simulink model "Test_World_3_cs"  (R2019a)
settings: Solver=FixedStepDiscrete  StartTime=0.0  StopTime=15  FixedStep=1/300  RelTol=1e-3
PreLoadFcn:
  | mbxruntime.callbacks.PreLoadFcn(bdroot);
  | check_NUTS_defined
  | model_closed = 0;
  | assignin('base',['model_closed_' bdroot],false);
PostLoadFcn:
  | mbxruntime.callbacks.PostLoadFcn(bdroot);
InitFcn:
  | mbxruntime.callbacks.InitFcn(bdroot);
StartFcn:
  | mbxruntime.callbacks.StartFcn(bdroot);
StopFcn:
  | mbxruntime.callbacks.StopFcn(bdroot);;
  | 
model workspace: external: MAT-File .\Test_World_3_cs_hws.mat (data not in the file)
undefined symbols (not defined in the file or in its folder): AngularVelocity, Clock_, Data, Data_SL_Info, DiscIntNeverNeededParam, Encoding, Encoding_SL_Info, Header, Height, InitImageOutputDir, LinearAcceleration, Orientation, Pose, Poses, Poses_SL_Info, Position, Step, Twist, Width
libraries: robotlib x26, simulink_extras x19, PreScanSimulinkLibrary x6, PBCSimulinkLibrary x5, dspindex x4, robotcorelib x2, sharedtransform x2, visionconversions x1, visionsinks x1
(part 2 of 5)

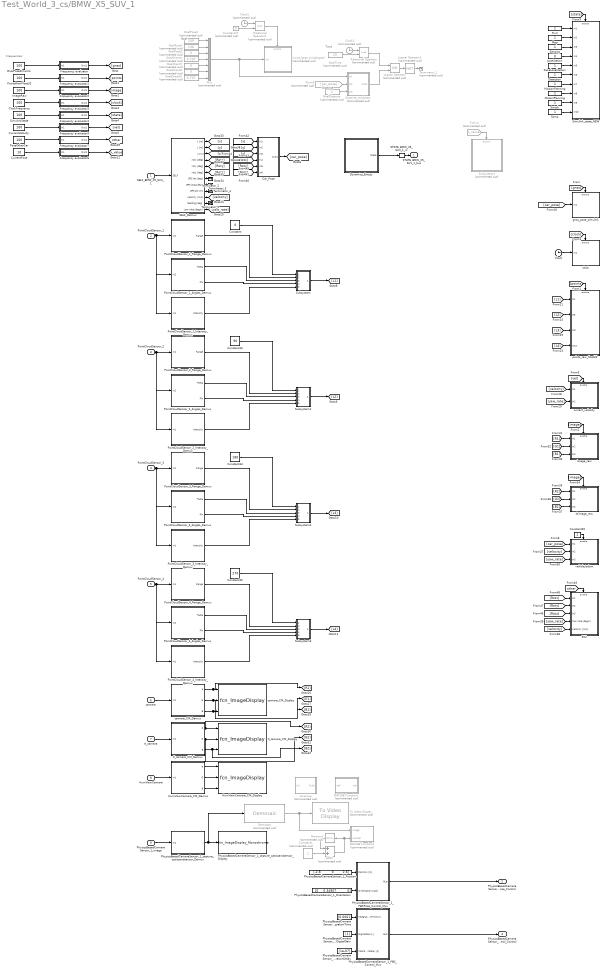
== system Test_World_3_cs/BMW_X5_SUV_1 ==
  note: Goal
  note: Distance
  note: Time
  note: Frequencies
  SELF_BMW_X5_SUV_1 : Inport  Tag=inport/SelfPort  OutDataTypeStr=Bus: PRESCAN_SELFSENSORDATA  PortDimensions=1  SampleTime=1/300  BusOutputAsStruct=on
  PointCloudSensor_1 : Inport  Tag=inport/PointCloudInport  Port=2  OutDataTypeStr=single  SampleTime=1/20  BusOutputAsStruct=on
  PointCloudSensor_2 : Inport  Tag=inport/PointCloudInport  Port=3  OutDataTypeStr=single  SampleTime=1/20  BusOutputAsStruct=on
  PointCloudSensor_3 : Inport  Tag=inport/PointCloudInport  Port=4  OutDataTypeStr=single  SampleTime=1/20  BusOutputAsStruct=on
  PointCloudSensor_4 : Inport  Tag=inport/PointCloudInport  Port=5  OutDataTypeStr=single  SampleTime=1/20  BusOutputAsStruct=on
  camera : Inport  Tag=inport/Camera/CameraSensor  Port=6  OutDataTypeStr=uint8  SampleTime=1/20  BusOutputAsStruct=on
  tl_camera : Inport  Tag=inport/Camera/CameraSensor  Port=7  OutDataTypeStr=uint8  SampleTime=1/20  BusOutputAsStruct=on
  HumViewCamera : Inport  Tag=inport/Camera/CameraSensor  Port=8  OutDataTypeStr=uint8  SampleTime=1/60  BusOutputAsStruct=on
  PhysicsBasedCameraSensor_1_image : Inport  Tag=inport/plugin/sfun_PBCOutput  Port=9  BusOutputAsStruct=on
  Add5 : Sum  Commented=on
  Car_Pose : Subsystem
  Clock : Clock
  Clock1 : Clock  Commented=on
  Clock2 : Clock  Commented=on
  ClockFrequency : Constant  Value=100
  Constant : Constant  Value=0  OutDataTypeStr=Inherit: Inherit via back propagation
  Constant1 : Constant  Commented=on  OutDataTypeStr=int32
  Constant20 : Constant
  Constant27 : Constant  Commented=on  Value=0
  Constant33 : Constant  Value=90  OutDataTypeStr=Inherit: Inherit via back propagation
  Constant34 : Constant  Value=180  OutDataTypeStr=Inherit: Inherit via back propagation
  Constant35 : Constant  Value=270  OutDataTypeStr=Inherit: Inherit via back propagation
  CurrentPose : Constant  Value=10
  CurrentVelocity : Constant  Value=100
  Demosaic : visionconversions/Demosaic  Commented=on  algorithm=Obsolete  algorithmActive=Gradient-corrected linear  alignment=BGGR  imagePorts=One multidimensional signal  roundingMode=Floor  overflowMode=on  prodOutputMode=Binary point scaling  prodOutputWordLength=32  prodOutputFracLength=10  prodOutputSlope=2^-10  accumSlope=2^-10
      settings: SourceProductName=Computer Vision Toolbox  SourceProductBaseCode=VP
  Detection : Constant
  Distance_evaluator : Subsystem  Commented=on
  Dynamics_Empty : Subsystem  Tag=Dynamics_Empty
      mask Help: eval('openHelp(202)')
      mask Display: port_label('output', 1, 'State');text(0,0,' Empty\n')
  FakeLocalization : Constant
  Frequency evaluator : Subsystem
  Frequency evaluator1 : Subsystem
  Frequency evaluator2 : Subsystem
  Frequency evaluator3 : Subsystem
  Frequency evaluator4 : Subsystem
  Frequency evaluator5 : Subsystem
  Frequency evaluator6 : Subsystem
  Frequency evaluator7 : Subsystem
  From4 : From  Commented=on  GotoTag=x_value
  From6 : From  Commented=on  GotoTag=car_pose
  GnssPoseSimulink : Constant  Value=100
  GoalDistance : Constant  Commented=on  Value=2
  GoalOrientW : Constant  Commented=on  Value=0.707
  GoalOrientX : Constant  Commented=on  Value=0.707
  GoalOrientY : Constant  Commented=on  Value=0
  GoalOrientZ : Constant  Commented=on  Value=0
  GoalPoseX : Constant  Commented=on  Value=249
  GoalPoseY : Constant  Commented=on  Value=136
  GoalPoseZ : Constant  Commented=on  Value=0
  GoalTime : Constant  Commented=on  Value=10
  HumViewCamera_CM_Demux : Subsystem  Tag=demux/Camera/Color  mask{SensorName=HumViewCamera, hres=1871, vres=1080}
      mask prompts: SensorName "Sensor Name"; hres "Horizontal Resolution"; vres "Vertical Resolution"
      mask Help: eval('openHelp(457)')
      mask Display:
      | fprintf('MONO CAMERA:\n Color\n %s \n %d x %d px',SensorName,hres,vres)
      | port_label('output',1,'R')
      | port_label('output',2,'G')
      | port_label('output',3,'B')
  HumViewCamera_CM_Display : M-S-Function  Tag=CameraSensor_Color_Display  InitFcn=InitImageOutputDir(gcb);  FunctionName=fcn_ImageDisplay  Parameters=SensorName EnableDisplay EnablePosition DisplayPosition FigureHandle SaveResults BitmapFormat TempOutputDir CameraType DataType  mask(PreScan Color Display Block){SensorName=HumViewCamera, EnableDisplay=on, EnablePosition=off, DisplayPosition=[10 10 1871 1080], FigureHandle=904007, SaveResults=off, Format=PNG, TempOutputDir=Results/SimResults_20190712_170005/HumViewCamera, CameraType=Mono, DataType=uint8}
      mask prompts: SensorName "User Specified: Title of Display"; EnableDisplay "Active"; EnablePosition "Set Display window position"; DisplayPosition "Display window position [xpos ypos width height]"; FigureHandle "Unique Handle"; SaveResults "Save results"; TempOutputDir "OutputDir"; CameraType "Camera Type"; DataType "Image Data Type"
      mask help: This block displays the RGB output of a PreScan camera sensor.
      mask init:
      | if EnableDisplay
      |     EnableString='';
      |     EnableColor='gray';
      | else
      |     EnableString='INACTIVE';
      |     EnableColor='red';
      | end
      | switch Format
      |     case 1
      |         BitmapFormat = 'png';
      |     case 2
      |         BitmapFormat = 'bmp';
      |     case 3
      |         BitmapFormat = 'jpg';
      | end 
      | if CameraType==1
      |     CameraTypeName='MONO';
      |     PortNumber=0;
      | else
      |     CameraTypeName='STEREO';
      |     PortNumber=3;
      | end
      settings: CopyFcn=CopyFcnDisplay  DeleteFcn=PreScanBlockDeleteFcn;  ModelCloseFcn=fcn_ImageDisplay_ModelCloseFcn
      mask Help: eval('openHelp(457)')
      mask Callback EnablePosition:
      | MV=get_param(gcb,'MaskVisibilities');
      | if strcmp(get_param(gcb,'EnablePosition'),'on')
      |     MV{4}='on';
      | else
      |     MV{4}='off';
      | end
      | set_param(gcb,'MaskVisibilities',MV);
      | clear MV;
      mask TypeOptions Format: PNG | BMP | JPG
      mask TypeOptions CameraType: Mono | Stereo
      mask TypeOptions DataType: uint8 | single
      mask Display:
      | color(EnableColor);
      | fprintf('%s\n DISPLAY:\n Color \n %s',EnableString,SensorName)
      | port_label('input',1,'R')
      | port_label('input',2,'G')
      | port_label('input',3,'B')
      | port_label('input',PortNumber+1,'R')
      | port_label('input',PortNumber+2,'G')
      | port_label('input',PortNumber+3,'B')
  IMU : Subsystem
  ImageRaw : Constant  Value=100
  Localization : Constant  Value=0
  Logical Operator : Logic  Commented=on  Operator=OR  AllPortsSameDT=off  OutDataTypeStr=boolean
  Logical Operator1 : Logic  Commented=on  Operator=NOT  AllPortsSameDT=off  OutDataTypeStr=boolean
  MATLAB Function1 : MATLAB Function  Commented=on  TreatAsAtomicUnit=on
  MATLAB Function2 : MATLAB Function  Commented=on  TreatAsAtomicUnit=on
  Map : Constant
  Memory2 : Memory  Commented=on  InheritSampleTime=on
  MissionPlanning : Constant
  MotionPlanning : Constant
  Mux : Mux  Commented=on  Inputs=7
  PhysicsBasedCameraSensor_1_DigitalGain : Constant  Tag=PhysicsBasedCameraSensor_1_DigitalGain  Value=[1]
  PhysicsBasedCameraSensor_1_IntegrationTime : Constant  Tag=PhysicsBasedCameraSensor_1_IntegrationTime  Value=[0.0001]
  PhysicsBasedCameraSensor_1_InterRowIntegrationDelay : Constant  Tag=PhysicsBasedCameraSensor_1_InterRowIntegrationDelay  Value=[1e-07]
  PhysicsBasedCameraSensor_1_Orientation : Constant  Tag=PhysicsBasedCameraSensor_1_Orientation  Value="[0     0.34907           0]"
  PhysicsBasedCameraSensor_1_PBCPose_Control_Mux : Subsystem  Tag=mux/plugin/PBC_TA
  PhysicsBasedCameraSensor_1_PBC_Control_Mux : Subsystem  Tag=mux/plugin/PBC_ControlSignalsBasic
  PhysicsBasedCameraSensor_1_Position : Constant  Tag=PhysicsBasedCameraSensor_1_Position  Value="[-2.8           0         2.6]"
  PhysicsBasedCameraSensor_1_capture_opticsandsensor_Demux : Subsystem  Tag=demux/Camera/Monochrome  mask{SensorName=PhysicsBasedCameraSensor_1, hres=1920, vres=1080}
      mask prompts: SensorName "Sensor Name"; hres "Horizontal Resolution"; vres "Vertical Resolution"
      mask Help: eval('openHelp(457)')
      mask Display:
      | fprintf('MONO CAMERA:\n Monochrome\n %s \n %d x %d px',SensorName,hres,vres)
      | port_label('output',1,'I')
  PhysicsBasedCameraSensor_1_capture_opticsandsensor_Display : M-S-Function  Tag=CameraSensor_Monochrome_Display  InitFcn=InitImageOutputDir(gcb);  FunctionName=fcn_ImageDisplay_Monochrome  Parameters=SensorName EnableDisplay EnablePosition DisplayPosition FigureHandle SaveResults BitmapFormat TempOutputDir CameraType DataType MaxValue  mask(PreScan Monochrome Display Block){SensorName=PhysicsBasedCameraSensor_1_capture_opticsandsensor, EnableDisplay=on, EnablePosition=off, DisplayPosition=[10 10 1080 1920], FigureHandle=1, SaveResults=off, Format=PNG, TempOutputDir=0, CameraType=Mono, DataType=single, MaxValue=-1}
      mask prompts: SensorName "User Specified: Title of Display"; EnableDisplay "Active"; EnablePosition "Set Display window position"; DisplayPosition "Display window position [xpos ypos width height]"; FigureHandle "Unique handle"; SaveResults "Save results"; TempOutputDir "OutputDir"; CameraType "Camera Type"; DataType "Image Data Type"; MaxValue "Maximum Value"
      mask help: This block displays the Monochrome output of a PreScan camera sensor.
      mask init:
      | if EnableDisplay
      |     EnableString='';
      |     EnableColor='gray';
      | else
      |     EnableString='INACTIVE';
      |     EnableColor='red';
      | end
      | switch Format
      |     case 1
      |         BitmapFormat = 'png';
      |     case 2
      |         BitmapFormat = 'bmp';
      |     case 3
      |         BitmapFormat = 'jpg';
      | end
      | if CameraType==1
      |     CameraTypeName='MONO';
      |     PortNumber=0;
      | else
      |     CameraTypeName='STEREO';
      |     PortNumber=1;
      | end
      settings: CopyFcn=CopyFcnDisplay  DeleteFcn=PreScanBlockDeleteFcn;  ModelCloseFcn=fcn_ImageDisplay_ModelCloseFcn
      mask Help: eval('openHelp(457)')
      mask Callback EnablePosition:
      | MV=get_param(gcb,'MaskVisibilities');
      | if strcmp(get_param(gcb,'EnablePosition'),'on')
      |     MV{4}='on';
      | else
      |     MV{4}='off';
      | end
      | set_param(gcb,'MaskVisibilities',MV);
      | clear MV;
      mask TypeOptions Format: PNG | BMP | JPG
      mask TypeOptions CameraType: Mono | Stereo
      mask TypeOptions DataType: uint8 | single | int32
      mask Callback DataType:
      | MV=get_param(gcb,'MaskVisibilities');
      | if strcmp(get_param(gcb,'DataType'),'int32')
      |     MV{6}='off';
      |     MV{7}='off';
      | else
      |     MV{6}='on';
      |     MV{7}='on';
      | end
      | set_param(gcb,'MaskVisibilities',MV);
      | clear MV;
      mask Display:
      | color(EnableColor);
      | fprintf('%s\n DISPLAY:\n Monochrome\n %s',EnableString,SensorName)
      | port_label('input',1,'I')
      | port_label('input',PortNumber+1,'I')
  PointCloudSensor_1_Angles_Demux : Subsystem  Tag=demux/PCS/Angles  mask{SensorName=PointCloudSensor_1, offset=225, hres=225, vres=16}
      mask prompts: SensorName "Sensor Name"; offset "Data Start"; hres "Horizontal Resolution"; vres "Vertical Resolution"
      mask Help: eval('openHelp(6400)')
      mask Display:
      | fprintf('Point Cloud:\n Data\n %s \n %d x %d px',SensorName,hres,vres)
      | port_label('output',1,'Theta')
      | port_label('output',2,'Phi')
  PointCloudSensor_1_Intensity_Demux : Subsystem  Tag=demux/PCS/Intensity  mask{SensorName=PointCloudSensor_1, offset=675, hres=225, vres=16}
      mask prompts: SensorName "Sensor Name"; offset "Data Start"; hres "Horizontal Resolution"; vres "Vertical Resolution"
      mask Help: eval('openHelp(6400)')
      mask Display:
      | fprintf('Point Cloud:\n Data\n %s \n %d x %d px',SensorName,hres,vres)
      | port_label('output',1,'Intensity')
  PointCloudSensor_1_Range_Demux : Subsystem  Tag=demux/PCS/Range  mask{SensorName=PointCloudSensor_1, offset=0, hres=225, vres=16}
      mask prompts: SensorName "Sensor Name"; offset "Data Start"; hres "Horizontal Resolution"; vres "Vertical Resolution"
      mask Help: eval('openHelp(6400)')
      mask Display:
      | fprintf('Point Cloud:\n Data\n %s \n %d x %d px',SensorName,hres,vres)
      | port_label('output',1,'Range')
  PointCloudSensor_2_Angles_Demux : Subsystem  Tag=demux/PCS/Angles  mask{SensorName=PointCloudSensor_2, offset=225, hres=225, vres=16}
      mask prompts: SensorName "Sensor Name"; offset "Data Start"; hres "Horizontal Resolution"; vres "Vertical Resolution"
      mask Help: eval('openHelp(6400)')
      mask Display:
      | fprintf('Point Cloud:\n Data\n %s \n %d x %d px',SensorName,hres,vres)
      | port_label('output',1,'Theta')
      | port_label('output',2,'Phi')
  PointCloudSensor_2_Intensity_Demux : Subsystem  Tag=demux/PCS/Intensity  mask{SensorName=PointCloudSensor_2, offset=675, hres=225, vres=16}
      mask prompts: SensorName "Sensor Name"; offset "Data Start"; hres "Horizontal Resolution"; vres "Vertical Resolution"
      mask Help: eval('openHelp(6400)')
      mask Display:
      | fprintf('Point Cloud:\n Data\n %s \n %d x %d px',SensorName,hres,vres)
      | port_label('output',1,'Intensity')
  PointCloudSensor_2_Range_Demux : Subsystem  Tag=demux/PCS/Range  mask{SensorName=PointCloudSensor_2, offset=0, hres=225, vres=16}
      mask prompts: SensorName "Sensor Name"; offset "Data Start"; hres "Horizontal Resolution"; vres "Vertical Resolution"
      mask Help: eval('openHelp(6400)')
      mask Display:
      | fprintf('Point Cloud:\n Data\n %s \n %d x %d px',SensorName,hres,vres)
      | port_label('output',1,'Range')
  PointCloudSensor_3_Angles_Demux : Subsystem  Tag=demux/PCS/Angles  mask{SensorName=PointCloudSensor_3, offset=225, hres=225, vres=16}
      mask prompts: SensorName "Sensor Name"; offset "Data Start"; hres "Horizontal Resolution"; vres "Vertical Resolution"
      mask Help: eval('openHelp(6400)')
      mask Display:
      | fprintf('Point Cloud:\n Data\n %s \n %d x %d px',SensorName,hres,vres)
      | port_label('output',1,'Theta')
      | port_label('output',2,'Phi')
  PointCloudSensor_3_Intensity_Demux : Subsystem  Tag=demux/PCS/Intensity  mask{SensorName=PointCloudSensor_3, offset=675, hres=225, vres=16}
      mask prompts: SensorName "Sensor Name"; offset "Data Start"; hres "Horizontal Resolution"; vres "Vertical Resolution"
      mask Help: eval('openHelp(6400)')
      mask Display:
      | fprintf('Point Cloud:\n Data\n %s \n %d x %d px',SensorName,hres,vres)
      | port_label('output',1,'Intensity')
  PointCloudSensor_3_Range_Demux : Subsystem  Tag=demux/PCS/Range  mask{SensorName=PointCloudSensor_3, offset=0, hres=225, vres=16}
      mask prompts: SensorName "Sensor Name"; offset "Data Start"; hres "Horizontal Resolution"; vres "Vertical Resolution"
      mask Help: eval('openHelp(6400)')
      mask Display:
      | fprintf('Point Cloud:\n Data\n %s \n %d x %d px',SensorName,hres,vres)
      | port_label('output',1,'Range')
  PointCloudSensor_4_Angles_Demux : Subsystem  Tag=demux/PCS/Angles  mask{SensorName=PointCloudSensor_4, offset=225, hres=225, vres=16}
      mask prompts: SensorName "Sensor Name"; offset "Data Start"; hres "Horizontal Resolution"; vres "Vertical Resolution"
      mask Help: eval('openHelp(6400)')
      mask Display:
      | fprintf('Point Cloud:\n Data\n %s \n %d x %d px',SensorName,hres,vres)
      | port_label('output',1,'Theta')
      | port_label('output',2,'Phi')
  PointCloudSensor_4_Intensity_Demux : Subsystem  Tag=demux/PCS/Intensity  mask{SensorName=PointCloudSensor_4, offset=675, hres=225, vres=16}
      mask prompts: SensorName "Sensor Name"; offset "Data Start"; hres "Horizontal Resolution"; vres "Vertical Resolution"
      mask Help: eval('openHelp(6400)')
      mask Display:
      | fprintf('Point Cloud:\n Data\n %s \n %d x %d px',SensorName,hres,vres)
      | port_label('output',1,'Intensity')
  PointCloudSensor_4_Range_Demux : Subsystem  Tag=demux/PCS/Range  mask{SensorName=PointCloudSensor_4, offset=0, hres=225, vres=16}
      mask prompts: SensorName "Sensor Name"; offset "Data Start"; hres "Horizontal Resolution"; vres "Vertical Resolution"
      mask Help: eval('openHelp(6400)')
      mask Display:
      | fprintf('Point Cloud:\n Data\n %s \n %d x %d px',SensorName,hres,vres)
      | port_label('output',1,'Range')
  PointsRawFloat32 : Constant  Value=100
  PoseOtherCar : Constant  Value=100
  Relational Operator : RelationalOperator  Commented=on  OutDataTypeStr=boolean  RndMeth=Simplest
  Relational Operator1 : RelationalOperator  Commented=on  Operator===  OutDataTypeStr=boolean  RndMeth=Simplest
  Rviz : Constant
  SELF_Demux : Subsystem  Tag=demux/SelfPort  mask(PreScan Demux Block:){}
      mask help:
      | The SELF port shows (state) information of the actor itself. The outputs are position in the experiment's axis system and the GPS coordinates, and the object's absolute velocity and compass heading.
      |
      | For more information, please click Help.
      settings: DeleteFcn=PreScanBlockDeleteFcn;
      mask Help: eval('openHelp(462)')
      mask Display:
      | port_label('output',1,'x [m]')
      | port_label('output',2,'y [m]')
      | port_label('output',3,'z [m]','texmode','on')
      | port_label('output',4,'Rotx [deg]','texmode','on')
      | port_label('output',5,'Roty [deg]','texmode','on')
      | port_label('output',6,'Rotz [deg]','texmode','on')
      | port_label('output',7,'GPS lat [deg]','texmode','on')
      | port_label('output',8,'GPS long [deg]','texmode','on')
      | port_label('output',9,'GPS alt [m]','texmode','on')
      | port_label('output',10,'Velocity [m/s]')
      | port_label('output',11,'Heading [deg]')
      | port_label('output',12,'Yaw rate [deg/s]')
  STATE_BMW_X5_SUV_1_rc : RateTransition  Tag=mux_rc/StatePort  OutPortSampleTimeOpt=Inherit
  Sensing : Constant
  SimulinkState : Constant  Value=100
  Simulink_state_NEW : Subsystem  TreatAsAtomicUnit=on
  Ssmp : Constant
  Subsystem : Subsystem
  Subsystem1 : Subsystem
  Subsystem2 : Subsystem
  Subsystem3 : Subsystem
  Subsystem4 : Subsystem  Commented=on
  Switch : Constant
  Terminator_1 : Terminator  Commented=on
  Terminator_{2..5} (4 alike) : Terminator
  To Video Display : visionsinks/To Video Display  Commented=on  windowSizeMode=Normal  openAtMdlStart=on  fullScreen=off  videoWindowX=0  videoWindowY=23  saveWindowSize=off  videoWindowWidth=1920  videoWindowHeight=1017  inputColorFormat=RGB  inputType=Obsolete  imagePorts=One multidimensional signal  OutputDevice=On-screen video monitor  dataOrg=Column-major  isWindowOpen=off
      settings: SourceProductName=Computer Vision Toolbox
  camera_CM_Demux : Subsystem  Tag=demux/Camera/Color  mask{SensorName=camera, hres=960, vres=720}
      mask prompts: SensorName "Sensor Name"; hres "Horizontal Resolution"; vres "Vertical Resolution"
      mask Help: eval('openHelp(457)')
      mask Display:
      | fprintf('MONO CAMERA:\n Color\n %s \n %d x %d px',SensorName,hres,vres)
      | port_label('output',1,'R')
      | port_label('output',2,'G')
      | port_label('output',3,'B')
  camera_CM_Display : M-S-Function  Tag=CameraSensor_Color_Display  InitFcn=InitImageOutputDir(gcb);  FunctionName=fcn_ImageDisplay  Parameters=SensorName EnableDisplay EnablePosition DisplayPosition FigureHandle SaveResults BitmapFormat TempOutputDir CameraType DataType  mask(PreScan Color Display Block){SensorName=camera, EnableDisplay=on, EnablePosition=off, DisplayPosition=[10 10 960 720], FigureHandle=904005, SaveResults=off, Format=PNG, TempOutputDir=0, CameraType=Mono, DataType=uint8}
      mask prompts: SensorName "User Specified: Title of Display"; EnableDisplay "Active"; EnablePosition "Set Display window position"; DisplayPosition "Display window position [xpos ypos width height]"; FigureHandle "Unique Handle"; SaveResults "Save results"; TempOutputDir "OutputDir"; CameraType "Camera Type"; DataType "Image Data Type"
      mask help: This block displays the RGB output of a PreScan camera sensor.
      mask init: same as Test_World_3_cs/BMW_X5_SUV_1/HumViewCamera_CM_Display
      settings: CopyFcn=CopyFcnDisplay  DeleteFcn=PreScanBlockDeleteFcn;  ModelCloseFcn=fcn_ImageDisplay_ModelCloseFcn
      mask Help: eval('openHelp(457)')
      mask Callback EnablePosition:
      | MV=get_param(gcb,'MaskVisibilities');
      | if strcmp(get_param(gcb,'EnablePosition'),'on')
      |     MV{4}='on';
      | else
      |     MV{4}='off';
      | end
      | set_param(gcb,'MaskVisibilities',MV);
      | clear MV;
      mask TypeOptions Format: PNG | BMP | JPG
      mask TypeOptions CameraType: Mono | Stereo
      mask TypeOptions DataType: uint8 | single
      mask Display:
      | color(EnableColor);
      | fprintf('%s\n DISPLAY:\n Color \n %s',EnableString,SensorName)
      | port_label('input',1,'R')
      | port_label('input',2,'G')
      | port_label('input',3,'B')
      | port_label('input',PortNumber+1,'R')
      | port_label('input',PortNumber+2,'G')
      | port_label('input',PortNumber+3,'B')
  clock : Subsystem
  current_velocity : Subsystem
  gnss_pose_simulink : Subsystem
  image_raw : Subsystem
  move_base_simple/goal : Subsystem  Commented=on  TreatAsAtomicUnit=on
  points_raw_float32 : Subsystem
  tl/image_raw : Subsystem
  tl_camera_CM_Demux : Subsystem  Tag=demux/Camera/Color  mask{SensorName=tl_camera, hres=960, vres=720}
      mask prompts: SensorName "Sensor Name"; hres "Horizontal Resolution"; vres "Vertical Resolution"
      mask Help: eval('openHelp(457)')
      mask Display:
      | fprintf('MONO CAMERA:\n Color\n %s \n %d x %d px',SensorName,hres,vres)
      | port_label('output',1,'R')
      | port_label('output',2,'G')
      | port_label('output',3,'B')
  tl_camera_CM_Display : M-S-Function  Tag=CameraSensor_Color_Display  InitFcn=InitImageOutputDir(gcb);  FunctionName=fcn_ImageDisplay  Parameters=SensorName EnableDisplay EnablePosition DisplayPosition FigureHandle SaveResults BitmapFormat TempOutputDir CameraType DataType  mask(PreScan Color Display Block){SensorName=tl_camera, EnableDisplay=on, EnablePosition=off, DisplayPosition=[10 10 960 720], FigureHandle=904006, SaveResults=off, Format=PNG, TempOutputDir=0, CameraType=Mono, DataType=uint8}
      mask prompts: SensorName "User Specified: Title of Display"; EnableDisplay "Active"; EnablePosition "Set Display window position"; DisplayPosition "Display window position [xpos ypos width height]"; FigureHandle "Unique Handle"; SaveResults "Save results"; TempOutputDir "OutputDir"; CameraType "Camera Type"; DataType "Image Data Type"
      mask help: This block displays the RGB output of a PreScan camera sensor.
      mask init: same as Test_World_3_cs/BMW_X5_SUV_1/HumViewCamera_CM_Display
      settings: CopyFcn=CopyFcnDisplay  DeleteFcn=PreScanBlockDeleteFcn;  ModelCloseFcn=fcn_ImageDisplay_ModelCloseFcn
      mask Help: eval('openHelp(457)')
      mask Callback EnablePosition:
      | MV=get_param(gcb,'MaskVisibilities');
      | if strcmp(get_param(gcb,'EnablePosition'),'on')
      |     MV{4}='on';
      | else
      |     MV{4}='off';
      | end
      | set_param(gcb,'MaskVisibilities',MV);
      | clear MV;
      mask TypeOptions Format: PNG | BMP | JPG
      mask TypeOptions CameraType: Mono | Stereo
      mask TypeOptions DataType: uint8 | single
      mask Display:
      | color(EnableColor);
      | fprintf('%s\n DISPLAY:\n Color \n %s',EnableString,SensorName)
      | port_label('input',1,'R')
      | port_label('input',2,'G')
      | port_label('input',3,'B')
      | port_label('input',PortNumber+1,'R')
      | port_label('input',PortNumber+2,'G')
      | port_label('input',PortNumber+3,'B')
  tonemap : Subsystem  Commented=on
  vehicle/odom : Subsystem
  STATE_BMW_X5_SUV_1_bus : Outport  Tag=outport/StatePort  OutDataTypeStr=Bus: PRESCAN_STATEACTUATORDATA  PortDimensions=1  SampleTime=1/300
  PhysicsBasedCameraSensor_1_PBCPose_Control : Outport  Tag=outport/plugin/sfun_PBCPose  Port=2  OutDataTypeStr=Bus: PRESCAN_PBCPOSE_DATA  PortDimensions=1  SampleTime=0.05
  PhysicsBasedCameraSensor_1_PBCControl_Control : Outport  Tag=outport/plugin/sfun_PBCControl  Port=3  OutDataTypeStr=Bus: PRESCAN_PBCCONTROL_DATA  PortDimensions=1  SampleTime=0.05
  tag scope: other=global, x_value=global
  wires:
  Car_Pose/1(Out1) -> [car_pose]
  [x] -> Car_Pose/1(In1)
  [y] -> Car_Pose/2(In2)
  [z] -> Car_Pose/3(In3)
  [Rotx] -> Car_Pose/4(In4)
  [Roty] -> Car_Pose/5(In5)
  [Rotz] -> Car_Pose/6(In6)
  Clock/1 -> clock/1(In1)
  [clock] -> clock/Enable
  Clock1/1 -> Relational Operator/1
  Relational Operator/1 -> Logical Operator/1
  Logical Operator/1 -> Logical Operator1/1
  Distance_evaluator/1(Out1) -> Logical Operator/2
  Mux/1 -> Distance_evaluator/1(In1), move_base_simple/goal/1(In1)
  Relational Operator1/1 -> move_base_simple/goal/Enable
  Clock2/1 -> Relational Operator1/1
  Constant27/1 -> Relational Operator1/2
  GoalPoseX/1 -> Mux/1
  GoalPoseY/1 -> Mux/2
  GoalPoseZ/1 -> Mux/3
  GoalOrientX/1 -> Mux/4
  GoalOrientY/1 -> Mux/5
  GoalOrientZ/1 -> Mux/6
  GoalOrientW/1 -> Mux/7
  From6/1 -> Distance_evaluator/2(In2)
  GoalDistance/1 -> Distance_evaluator/3(In3)
  GoalTime/1 -> Relational Operator/2
  Constant/1 -> Subsystem/1(In1)
  Subsystem/1(Out1) -> [L1]
  PointCloudSensor_1_Range_Demux/1(Range) -> Subsystem/2(In2)
  PointCloudSensor_1_Angles_Demux/1(Theta) -> Subsystem/3(In3)
  PointCloudSensor_1_Angles_Demux/2(Phi) -> Subsystem/4(In4)
  PointCloudSensor_1_Intensity_Demux/1(Intensity) -> Subsystem/5(In5)
  FakeLocalization/1 -> Simulink_state_NEW/5(In5)
  Rviz/1 -> Simulink_state_NEW/1(In1)
  Map/1 -> Simulink_state_NEW/2(In2)
  Sensing/1 -> Simulink_state_NEW/3(In3)
  Localization/1 -> Simulink_state_NEW/4(In4)
  Detection/1 -> Simulink_state_NEW/6(In6)
  MissionPlanning/1 -> Simulink_state_NEW/7(In7)
  MotionPlanning/1 -> Simulink_state_NEW/8(In8)
  Switch/1 -> Simulink_state_NEW/9(In9)
  Ssmp/1 -> Simulink_state_NEW/10(In10)
  [state] -> Simulink_state_NEW/Enable
  Constant20/1 -> vehicle/odom/Enable
  [car_pose] -> vehicle/odom/1(In1)
  [velocity] -> vehicle/odom/2(In2)
  [yaw_rate] -> vehicle/odom/3(In3)
  GnssPoseSimulink/1 -> Frequency evaluator/1(In1)
  Frequency evaluator/1(Out1) -> [gnss]
  PointsRawFloat32/1 -> Frequency evaluator1/1(In1)
  Frequency evaluator1/1(Out1) -> [points]
  ImageRaw/1 -> Frequency evaluator2/1(In1)
  Frequency evaluator2/1(Out1) -> [image]
  ClockFrequency/1 -> Frequency evaluator3/1(In1)
  Frequency evaluator3/1(Out1) -> [clock]
  SimulinkState/1 -> Frequency evaluator4/1(In1)
  Frequency evaluator4/1(Out1) -> [state]
  CurrentVelocity/1 -> Frequency evaluator5/1(In1)
  Frequency evaluator5/1(Out1) -> [vel]
  PoseOtherCar/1 -> Frequency evaluator7/1(In1)
  Frequency evaluator7/1(Out1) -> [other]
  Constant33/1 -> Subsystem1/1(In1)
  Subsystem1/1(Out1) -> [L2]
  PointCloudSensor_2_Range_Demux/1(Range) -> Subsystem1/2(In2)
  PointCloudSensor_2_Angles_Demux/1(Theta) -> Subsystem1/3(In3)
  PointCloudSensor_2_Angles_Demux/2(Phi) -> Subsystem1/4(In4)
  PointCloudSensor_2_Intensity_Demux/1(Intensity) -> Subsystem1/5(In5)
  Constant34/1 -> Subsystem2/1(In1)
  Subsystem2/1(Out1) -> [L3]
  PointCloudSensor_3_Range_Demux/1(Range) -> Subsystem2/2(In2)
  PointCloudSensor_3_Angles_Demux/1(Theta) -> Subsystem2/3(In3)
  PointCloudSensor_3_Angles_Demux/2(Phi) -> Subsystem2/4(In4)
  PointCloudSensor_3_Intensity_Demux/1(Intensity) -> Subsystem2/5(In5)
  Constant35/1 -> Subsystem3/1(In1)
  Subsystem3/1(Out1) -> [L4]
  PointCloudSensor_4_Range_Demux/1(Range) -> Subsystem3/2(In2)
  PointCloudSensor_4_Angles_Demux/1(Theta) -> Subsystem3/3(In3)
  PointCloudSensor_4_Angles_Demux/2(Phi) -> Subsystem3/4(In4)
  PointCloudSensor_4_Intensity_Demux/1(Intensity) -> Subsystem3/5(In5)
  [gnss] -> gnss_pose_simulink/Enable
  [car_pose] -> gnss_pose_simulink/1(In1)
  [points] -> points_raw_float32/Enable
  [L1] -> points_raw_float32/1(In1)
  [L2] -> points_raw_float32/2(In5)
  [L3] -> points_raw_float32/3(In9)
  [L4] -> points_raw_float32/4(In13)
  [image] -> image_raw/Enable
  [R1] -> image_raw/1(In1)
  [G1] -> image_raw/2(In2)
  [B1] -> image_raw/3(In3)
  [velocity] -> current_velocity/1(In1)
  [yaw_rate] -> current_velocity/2(In2)
  [vel] -> current_velocity/Enable
  [image] -> tl/image_raw/Enable
  [R2] -> tl/image_raw/1(In1)
  [G2] -> tl/image_raw/2(In2)
  [B2] -> tl/image_raw/3(In3)
  [velocity] -> IMU/5(Velocity [m/s])
  [Rotx] -> IMU/1(In1)
  [Roty] -> IMU/2(In2)
  [Rotz] -> IMU/3(In3)
  [yaw_rate] -> IMU/4(Yaw rate [deg/s])
  [other] -> IMU/Enable
  SELF_Demux/10(velocity [m/s]) -> [velocity]
  SELF_Demux/12(yaw rate [deg/s]) -> [yaw_rate]
  camera_CM_Demux/1(R) -> [R1], camera_CM_Display/1
  camera_CM_Demux/2(G) -> [G1], camera_CM_Display/2
  camera_CM_Demux/3(B) -> [B1], camera_CM_Display/3
  tl_camera_CM_Demux/1(R) -> [R2], tl_camera_CM_Display/1
  tl_camera_CM_Demux/2(G) -> [G2], tl_camera_CM_Display/2
  tl_camera_CM_Demux/3(B) -> [B2], tl_camera_CM_Display/3
  SELF_Demux/1(x [m]) -> [x]
  SELF_Demux/6(rotz [deg]) -> [Rotz]
  SELF_Demux/5(roty [deg]) -> [Roty]
  SELF_Demux/4(rotx [deg]) -> [Rotx]
  SELF_Demux/3(z [m]) -> [z]
  SELF_Demux/2(y [m]) -> [y]
  Frequency evaluator6/1(Out1) -> [x_value]
  CurrentPose/1 -> Frequency evaluator6/1(In1)
  From4/1 -> Subsystem4/Enable
  PhysicsBasedCameraSensor_1_capture_opticsandsensor_Demux/1(I) -> Demosaic/1, PhysicsBasedCameraSensor_1_capture_opticsandsensor_Display/1
  Add5/1 -> Memory2/1, MATLAB Function2/2(counter)
  Memory2/1 -> Add5/1
  Constant1/1 -> Add5/2
  Demosaic/1 -> MATLAB Function2/1(image), To Video Display/1
  STATE_BMW_X5_SUV_1_rc/1 -> STATE_BMW_X5_SUV_1_bus/1
  SELF_BMW_X5_SUV_1/1 -> SELF_Demux/1(SELF)
  PointCloudSensor_1/1 -> PointCloudSensor_1_Range_Demux/1(In1), PointCloudSensor_1_Angles_Demux/1(In2), PointCloudSensor_1_Intensity_Demux/1(In1)
  PointCloudSensor_2/1 -> PointCloudSensor_2_Range_Demux/1(In1), PointCloudSensor_2_Angles_Demux/1(In2), PointCloudSensor_2_Intensity_Demux/1(In1)
  PointCloudSensor_3/1 -> PointCloudSensor_3_Range_Demux/1(In1), PointCloudSensor_3_Angles_Demux/1(In2), PointCloudSensor_3_Intensity_Demux/1(In1)
  PointCloudSensor_4/1 -> PointCloudSensor_4_Range_Demux/1(In1), PointCloudSensor_4_Angles_Demux/1(In2), PointCloudSensor_4_Intensity_Demux/1(In1)
  camera/1 -> camera_CM_Demux/1(In1)
  tl_camera/1 -> tl_camera_CM_Demux/1(In1)
  HumViewCamera/1 -> HumViewCamera_CM_Demux/1(In1)
  HumViewCamera_CM_Demux/1(R) -> HumViewCamera_CM_Display/1
  HumViewCamera_CM_Demux/2(G) -> HumViewCamera_CM_Display/2
  HumViewCamera_CM_Demux/3(B) -> HumViewCamera_CM_Display/3
  Dynamics_Empty/1(State) -> STATE_BMW_X5_SUV_1_rc/1
  PhysicsBasedCameraSensor_1_image/1 -> PhysicsBasedCameraSensor_1_capture_opticsandsensor_Demux/1(In1)
  PhysicsBasedCameraSensor_1_PBCPose_Control_Mux/1(Bus) -> PhysicsBasedCameraSensor_1_PBCPose_Control/1
  PhysicsBasedCameraSensor_1_Position/1 -> PhysicsBasedCameraSensor_1_PBCPose_Control_Mux/1(Position [m])
  PhysicsBasedCameraSensor_1_Orientation/1 -> PhysicsBasedCameraSensor_1_PBCPose_Control_Mux/2(Orientation [rad])
  PhysicsBasedCameraSensor_1_PBC_Control_Mux/1(Bus) -> PhysicsBasedCameraSensor_1_PBCControl_Control/1
  PhysicsBasedCameraSensor_1_IntegrationTime/1 -> PhysicsBasedCameraSensor_1_PBC_Control_Mux/1(IntegrationTime [s])
  PhysicsBasedCameraSensor_1_DigitalGain/1 -> PhysicsBasedCameraSensor_1_PBC_Control_Mux/2(DigitalGain [-])
  PhysicsBasedCameraSensor_1_InterRowIntegrationDelay/1 -> PhysicsBasedCameraSensor_1_PBC_Control_Mux/3(InterRowIntegrationDelay [s])
  Logical Operator1/1 -> Terminator_1/1
  SELF_Demux/7(GPS lat [deg]) -> Terminator_2/1
  SELF_Demux/8(GPS long [deg]) -> Terminator_3/1
  SELF_Demux/9(GPS alt [m]) -> Terminator_4/1
  SELF_Demux/11(heading [deg]) -> Terminator_5/1

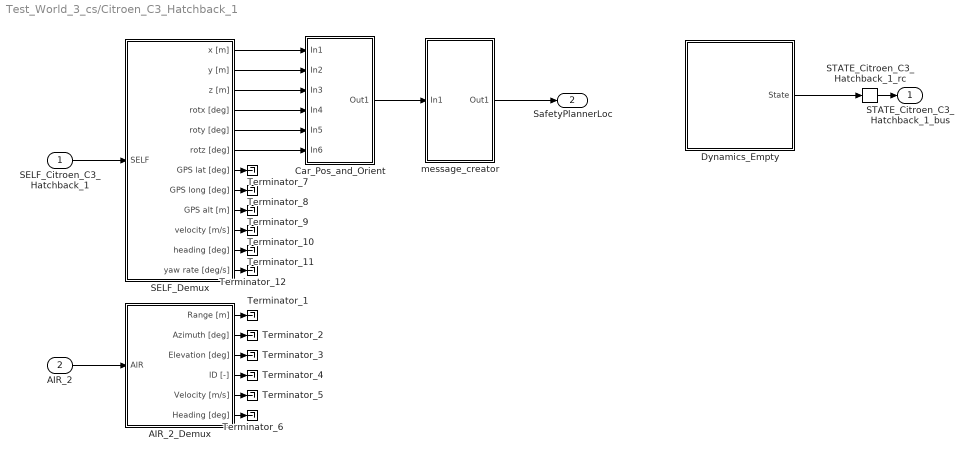
== system Test_World_3_cs/Citroen_C3_Hatchback_1 ==
  SELF_Citroen_C3_Hatchback_1 : Inport  Tag=inport/SelfPort  OutDataTypeStr=Bus: PRESCAN_SELFSENSORDATA  PortDimensions=1  SampleTime=1/300  BusOutputAsStruct=on
  AIR_2 : Inport  Tag=inport/AIR  Port=2  OutDataTypeStr=Bus: PRESCAN_AIRSENSORMESSAGE  PortDimensions=1  SampleTime=1/300  BusOutputAsStruct=on
  AIR_2_Demux : Subsystem  Tag=demux/AIR  mask(PreScan Demux Block: AIR){DetectionType=BBox, detectableObjects=1}
      mask prompts: DetectionType "Detection Type"; detectableObjects "Max. detectable objects"
      mask help:
      | The Actor Information Receiver sensor provides a fast, simple and generic detection solution which is not tied up to a specific technology and can be used for scenarios in which a simple sensor is needed.
      |
      | For more information, please click Help.
      mask init:
      | switch DetectionType
      |     case 1
      |         DetectionTypeStr = 'Center';
      |     case 2
      |         DetectionTypeStr = 'BBox';
      |     case 3
      |         DetectionTypeStr = 'CoG';
      |     otherwise
      |         DetectionTypeStr = 'Unknown';
      | end
      settings: DeleteFcn=PreScanBlockDeleteFcn;
      mask Help: eval('openHelp(413)')
      mask TypeOptions DetectionType: Center | BBox | CoG
      mask Display:
      | disp(char('Det. type:         ',['{\it',DetectionTypeStr,'}']),'texmode','on')
      | port_label('output',1,'Range [m]')
      | port_label('output',2,'{\theta} [deg]','texmode','on')
      | port_label('output',3,'{\phi} [deg]','texmode','on')
      | port_label('output',4,'ID [-]','texmode','on')
      | port_label('output',5,'Velocity [m/s]','texmode','on')
      | port_label('output',6,'Heading [deg]','texmode','on')
  Car_Pos_and_Orient : Subsystem
  Dynamics_Empty : Subsystem  Tag=Dynamics_Empty
      mask Help: eval('openHelp(202)')
      mask Display: port_label('output', 1, 'State');text(0,0,' Empty\n')
  SELF_Demux : Subsystem  Tag=demux/SelfPort  mask(PreScan Demux Block:){}
      mask help:
      | The SELF port shows (state) information of the actor itself. The outputs are position in the experiment's axis system and the GPS coordinates, and the object's absolute velocity and compass heading.
      |
      | For more information, please click Help.
      settings: DeleteFcn=PreScanBlockDeleteFcn;
      mask Help: eval('openHelp(462)')
      mask Display:
      | port_label('output',1,'x [m]')
      | port_label('output',2,'y [m]')
      | port_label('output',3,'z [m]','texmode','on')
      | port_label('output',4,'Rotx [deg]','texmode','on')
      | port_label('output',5,'Roty [deg]','texmode','on')
      | port_label('output',6,'Rotz [deg]','texmode','on')
      | port_label('output',7,'GPS lat [deg]','texmode','on')
      | port_label('output',8,'GPS long [deg]','texmode','on')
      | port_label('output',9,'GPS alt [m]','texmode','on')
      | port_label('output',10,'Velocity [m/s]')
      | port_label('output',11,'Heading [deg]')
      | port_label('output',12,'Yaw rate [deg/s]')
  STATE_Citroen_C3_Hatchback_1_rc : RateTransition  Tag=mux_rc/StatePort  OutPortSampleTimeOpt=Inherit
  Terminator_{1..12} (12 alike) : Terminator
  message_creator : Subsystem
  STATE_Citroen_C3_Hatchback_1_bus : Outport  Tag=outport/StatePort  OutDataTypeStr=Bus: PRESCAN_STATEACTUATORDATA  PortDimensions=1  SampleTime=1/300
  SafetyPlannerLoc : Outport  Port=2
  wires:
  Car_Pos_and_Orient/1(Out1) -> message_creator/1(In1)
  message_creator/1(Out1) -> SafetyPlannerLoc/1
  SELF_Demux/1(x [m]) -> Car_Pos_and_Orient/1(In1)
  SELF_Demux/2(y [m]) -> Car_Pos_and_Orient/2(In2)
  SELF_Demux/3(z [m]) -> Car_Pos_and_Orient/3(In3)
  SELF_Demux/4(rotx [deg]) -> Car_Pos_and_Orient/4(In4)
  SELF_Demux/5(roty [deg]) -> Car_Pos_and_Orient/5(In5)
  SELF_Demux/6(rotz [deg]) -> Car_Pos_and_Orient/6(In6)
  STATE_Citroen_C3_Hatchback_1_rc/1 -> STATE_Citroen_C3_Hatchback_1_bus/1
  SELF_Citroen_C3_Hatchback_1/1 -> SELF_Demux/1(SELF)
  AIR_2/1 -> AIR_2_Demux/1(AIR)
  Dynamics_Empty/1(State) -> STATE_Citroen_C3_Hatchback_1_rc/1
  AIR_2_Demux/1(Range [m]) -> Terminator_1/1
  AIR_2_Demux/2(Azimuth [deg]) -> Terminator_2/1
  AIR_2_Demux/3(Elevation [deg]) -> Terminator_3/1
  AIR_2_Demux/4(ID [-]) -> Terminator_4/1
  AIR_2_Demux/5(Velocity [m/s]) -> Terminator_5/1
  AIR_2_Demux/6(Heading [deg]) -> Terminator_6/1
  SELF_Demux/7(GPS lat [deg]) -> Terminator_7/1
  SELF_Demux/8(GPS long [deg]) -> Terminator_8/1
  SELF_Demux/9(GPS alt [m]) -> Terminator_9/1
  SELF_Demux/10(velocity [m/s]) -> Terminator_10/1
  SELF_Demux/11(heading [deg]) -> Terminator_11/1
  SELF_Demux/12(yaw rate [deg/s]) -> Terminator_12/1

== system Test_World_3_cs/Controller ==
  Terminator : Terminator
  sfun_Controller : S-Function  FunctionName=sfun_Controller  Parameters=SParameter1, SParameter2, SParameter3, SParameter4, SParameter5, SParameter6, SParameter7, SParameter8, SParameter9, SParameter10, SampleTime  SFunctionDeploymentMode=off  EnableBusSupport=off  mask(Legacy Function){SFunctionSpec=void prescan_outputFcn(void** work1, PRESCAN_CONTROLLERDATA y1[1]), SParameter1=uint8([ExperimentFile 0]), SParameter2=uint8([ModelDepo 0]), SParameter3=uint8([ControllerOptions 0]), SParameter4=RTmode, SParameter5=PreScanExecutionMode, SParameter6=ControlMode, SParameter7=ControllerCount, SParameter8=ControllerIndex, SParameter9=uint8([SimulationMode 0]), SParameter10=uint8([TargetName 0]), SampleTime=TimeStep, ShowSpec=on}
      mask prompts: SParameter1 "P1:"; SParameter2 "P2:"; SParameter3 "P3:"; SParameter4 "P4:"; SParameter5 "P5:"; SParameter6 "P6:"; SParameter7 "P7:"; SParameter8 "P8:"; SParameter9 "P9:"; SParameter10 "P10:"; SampleTime "Sample time (-1 for inherited):"; ShowSpec "Display function specification"
      mask help:
      | This block allows you to call the legacy functions specified by the following Legacy Code Tool definition:
      | def.SFunctionName = 'sfun_Controller';
      | def.OutputFcnSpec = 'void prescan_outputFcn(void** work1, PRESCAN_CONTROLLERDATA y1[1])';
      | def.StartFcnSpec = 'void prescan_startFcn(void ** work1, uint8 p1[], uint8 p2[], uint8 p3[], double p4, double p5, double p6, double p7, double p8, uint8 p9[], uint8 p10[])';
      | def.TerminateFcnSpec = 'void prescan_terminateFcn(void** work1)';
      | def.HeaderFiles = {'prescan_controller_data.h', 'prescan_SFunLibrary.h', 'prescan_CreateLogHandler.h', 'prescan_CreateErrorHandler.h', 'prescan_modify.h', 'ModuleDLL.h'};
      | def.SourceFiles = {'prescan_MexLogHandler.c', 'prescan_SimStructErrorHandler.c', 'prescan_LogHandler.c', 'prescan_ErrorHandler.c', 'prescan_Modify.c'};
      | def.HostLibFiles = {'sensorinterfaced.lib'};
      | def.TargetLibFiles = {'sensorinterfaced.so'};
      | def.IncPaths = {'.', 'C:\projects\prescan\rt_vislibrary\vis\..\pimp\include\sensors\InterfaceRTW'};
      | def.SrcPaths = {'C:\projects\prescan\rt_vislibrary\vis\..\pimp\include\sensors\InterfaceRTW', 'C:\projects\prescan\rt_vislibrary\vis\..\pimp\include\sensors\InterfaceRTW\ccurrt'};
      | def.LibPaths = {'C:\\projects\\prescan\\vislibrary_build\lib'};
      | def.SampleTime = 'parameterized';
      mask Help: <p>This block was generated automatically by the Legacy Code Tool. For detailed help on this tool, call<a href="matlab:legacy_code('help')"> legacy_code('help')</a>.</p>
      mask Callback ShowSpec:
      | if strcmp(get_param(gcbh, 'ShowSpec'), 'on')
      |   set_param(gcbh, 'MaskDisplay', sprintf('fprintf(''%s'');', get_param(gcbh, 'SFunctionSpec')));
      | else
      |   set_param(gcbh, 'MaskDisplay', sprintf('fprintf(''%s'');', get_param(gcbh, 'FunctionName')));
      | end
      mask Display: fprintf('void prescan_outputFcn(void** work1, PRESCAN_CONTROLLERDATA y1[1])');
  wires:
  sfun_Controller/1 -> Terminator/1

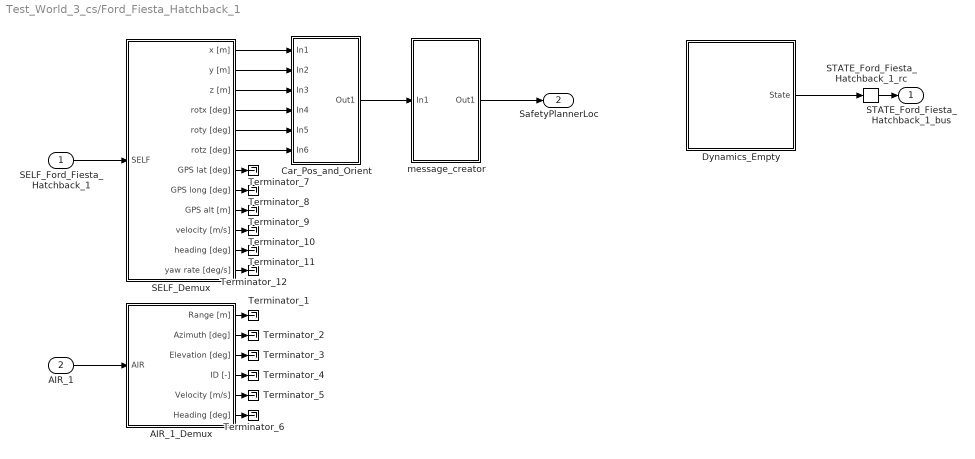
== system Test_World_3_cs/Ford_Fiesta_Hatchback_1 ==
  SELF_Ford_Fiesta_Hatchback_1 : Inport  Tag=inport/SelfPort  OutDataTypeStr=Bus: PRESCAN_SELFSENSORDATA  PortDimensions=1  SampleTime=1/300  BusOutputAsStruct=on
  AIR_1 : Inport  Tag=inport/AIR  Port=2  OutDataTypeStr=Bus: PRESCAN_AIRSENSORMESSAGE  PortDimensions=1  SampleTime=1/300  BusOutputAsStruct=on
  AIR_1_Demux : Subsystem  Tag=demux/AIR  mask(PreScan Demux Block: AIR){DetectionType=BBox, detectableObjects=1}
      mask prompts: DetectionType "Detection Type"; detectableObjects "Max. detectable objects"
      mask help:
      | The Actor Information Receiver sensor provides a fast, simple and generic detection solution which is not tied up to a specific technology and can be used for scenarios in which a simple sensor is needed.
      |
      | For more information, please click Help.
      mask init: same as Test_World_3_cs/Citroen_C3_Hatchback_1/AIR_2_Demux
      settings: DeleteFcn=PreScanBlockDeleteFcn;
      mask Help: eval('openHelp(413)')
      mask TypeOptions DetectionType: Center | BBox | CoG
      mask Display:
      | disp(char('Det. type:         ',['{\it',DetectionTypeStr,'}']),'texmode','on')
      | port_label('output',1,'Range [m]')
      | port_label('output',2,'{\theta} [deg]','texmode','on')
      | port_label('output',3,'{\phi} [deg]','texmode','on')
      | port_label('output',4,'ID [-]','texmode','on')
      | port_label('output',5,'Velocity [m/s]','texmode','on')
      | port_label('output',6,'Heading [deg]','texmode','on')
  Car_Pos_and_Orient : Subsystem
  Dynamics_Empty : Subsystem  Tag=Dynamics_Empty
      mask Help: eval('openHelp(202)')
      mask Display: port_label('output', 1, 'State');text(0,0,' Empty\n')
  SELF_Demux : Subsystem  Tag=demux/SelfPort  mask(PreScan Demux Block:){}
      mask help:
      | The SELF port shows (state) information of the actor itself. The outputs are position in the experiment's axis system and the GPS coordinates, and the object's absolute velocity and compass heading.
      |
      | For more information, please click Help.
      settings: DeleteFcn=PreScanBlockDeleteFcn;
      mask Help: eval('openHelp(462)')
      mask Display:
      | port_label('output',1,'x [m]')
      | port_label('output',2,'y [m]')
      | port_label('output',3,'z [m]','texmode','on')
      | port_label('output',4,'Rotx [deg]','texmode','on')
      | port_label('output',5,'Roty [deg]','texmode','on')
      | port_label('output',6,'Rotz [deg]','texmode','on')
      | port_label('output',7,'GPS lat [deg]','texmode','on')
      | port_label('output',8,'GPS long [deg]','texmode','on')
      | port_label('output',9,'GPS alt [m]','texmode','on')
      | port_label('output',10,'Velocity [m/s]')
      | port_label('output',11,'Heading [deg]')
      | port_label('output',12,'Yaw rate [deg/s]')
  STATE_Ford_Fiesta_Hatchback_1_rc : RateTransition  Tag=mux_rc/StatePort  OutPortSampleTimeOpt=Inherit
  Terminator_{1..12} (12 alike) : Terminator
  message_creator : Subsystem
  STATE_Ford_Fiesta_Hatchback_1_bus : Outport  Tag=outport/StatePort  OutDataTypeStr=Bus: PRESCAN_STATEACTUATORDATA  PortDimensions=1  SampleTime=1/300
  SafetyPlannerLoc : Outport  Port=2
  wires:
  Car_Pos_and_Orient/1(Out1) -> message_creator/1(In1)
  message_creator/1(Out1) -> SafetyPlannerLoc/1
  SELF_Demux/1(x [m]) -> Car_Pos_and_Orient/1(In1)
  SELF_Demux/2(y [m]) -> Car_Pos_and_Orient/2(In2)
  SELF_Demux/3(z [m]) -> Car_Pos_and_Orient/3(In3)
  SELF_Demux/4(rotx [deg]) -> Car_Pos_and_Orient/4(In4)
  SELF_Demux/5(roty [deg]) -> Car_Pos_and_Orient/5(In5)
  SELF_Demux/6(rotz [deg]) -> Car_Pos_and_Orient/6(In6)
  STATE_Ford_Fiesta_Hatchback_1_rc/1 -> STATE_Ford_Fiesta_Hatchback_1_bus/1
  SELF_Ford_Fiesta_Hatchback_1/1 -> SELF_Demux/1(SELF)
  AIR_1/1 -> AIR_1_Demux/1(AIR)
  Dynamics_Empty/1(State) -> STATE_Ford_Fiesta_Hatchback_1_rc/1
  AIR_1_Demux/1(Range [m]) -> Terminator_1/1
  AIR_1_Demux/2(Azimuth [deg]) -> Terminator_2/1
  AIR_1_Demux/3(Elevation [deg]) -> Terminator_3/1
  AIR_1_Demux/4(ID [-]) -> Terminator_4/1
  AIR_1_Demux/5(Velocity [m/s]) -> Terminator_5/1
  AIR_1_Demux/6(Heading [deg]) -> Terminator_6/1
  SELF_Demux/7(GPS lat [deg]) -> Terminator_7/1
  SELF_Demux/8(GPS long [deg]) -> Terminator_8/1
  SELF_Demux/9(GPS alt [m]) -> Terminator_9/1
  SELF_Demux/10(velocity [m/s]) -> Terminator_10/1
  SELF_Demux/11(heading [deg]) -> Terminator_11/1
  SELF_Demux/12(yaw rate [deg/s]) -> Terminator_12/1

== system Test_World_3_cs/HumViewCamera ==
  Sensor : S-Function  FunctionName=sfun_Camera  Parameters=sensorID, dataWidth, dataHeight, channelsPerImage, numberOfImages, timestep  SFunctionDeploymentMode=off  EnableBusSupport=off  mask(PreScan Source Block: Camera Sensor){sensorID=14458, dataWidth=1080, dataHeight=5613, channelsPerImage=3, numberOfImages=1, timestep=1/60}
      mask prompts: sensorID "Sensor ID"; dataWidth "Data width"; dataHeight "Data Height"; channelsPerImage "Channels per image"; numberOfImages "Number of images"; timestep "MATLAB timestep:"
      mask help: The Camera Sensor provides a color or monochrome image.
      mask Help: eval('openHelp(457)')
      mask Display: image(imread('CameraSensor.png'))
  HumViewCamera : Outport  Tag=outport/Camera/CameraSensor  OutDataTypeStr=uint8  SampleTime=1/60
  wires:
  Sensor/1 -> HumViewCamera/1

== system Test_World_3_cs/PhysicsBasedCameraSensor_1_PBCControl_Control ==
  PhysicsBasedCameraSensor_1_PBCControl_Control : Inport  Tag=inport/plugin/sfun_PBCControl  OutDataTypeStr=Bus: PRESCAN_PBCCONTROL_DATA  PortDimensions=1  SampleTime=0.05  BusOutputAsStruct=on
  Actuator : S-Function  LoadFcn=addpath 'C:/Program Files/Simcenter Prescan/Prescan_2019.1/Plugins/PBCameraPlugin/matlab';addpath 'C:/Program Files/Simcenter Prescan/Prescan_2019.1/Plugins/PBCameraPlugin/bin';load('PreScanPBCControlData.mat');  FunctionName=sfun_PBCControl  Parameters=sensorID, timestep  SFunctionDeploymentMode=off  EnableBusSupport=off  mask(Physics Based Camera plugin block){sensorID=0, timestep=0.05}
      mask prompts: sensorID "Sensor ID"; timestep "MATLAB timestep:"
      mask help: PBC Control I/O
      mask Help: eval('openHelp(6500)')
      mask Display: image(imread('ico_PBCControl.png'))
  wires:
  PhysicsBasedCameraSensor_1_PBCControl_Control/1 -> Actuator/1

== system Test_World_3_cs/PhysicsBasedCameraSensor_1_PBCPose_Control ==
  PhysicsBasedCameraSensor_1_PBCPose_Control : Inport  Tag=inport/plugin/sfun_PBCPose  OutDataTypeStr=Bus: PRESCAN_PBCPOSE_DATA  PortDimensions=1  SampleTime=0.05  BusOutputAsStruct=on
  Actuator : S-Function  LoadFcn=addpath 'C:/Program Files/Simcenter Prescan/Prescan_2019.1/Plugins/PBCameraPlugin/matlab';addpath 'C:/Program Files/Simcenter Prescan/Prescan_2019.1/Plugins/PBCameraPlugin/bin';load('PreScanPBCPoseData.mat');  FunctionName=sfun_PBCPose  Parameters=sensorID, timestep  SFunctionDeploymentMode=off  EnableBusSupport=off  mask(Physics Based Camera plugin block){sensorID=0, timestep=0.05}
      mask prompts: sensorID "Sensor ID"; timestep "MATLAB timestep:"
      mask help: PBC Control I/O
      mask Help: eval('openHelp(6500)')
      mask Display: image(imread('ico_PBCControl.png'))
  wires:
  PhysicsBasedCameraSensor_1_PBCPose_Control/1 -> Actuator/1

== system Test_World_3_cs/PhysicsBasedCameraSensor_1_image ==
  Sensor : S-Function  FunctionName=sfun_PBCOutput  Parameters=cameraID, dataWidth, dataHeight, timestepMask  SFunctionDeploymentMode=off  EnableBusSupport=off  mask(Physics Based Camera plugin block){cameraID=0, dataWidth=1080, dataHeight=1920, timestepMask=0.05}
      mask prompts: cameraID "Camera ID:"; dataWidth "Data width"; dataHeight "Data height"; timestepMask "MATLAB timestep:"
      mask help: Physics Based Camera image
      mask Help: eval('openHelp(6500)')
      mask Display: image(imread('ico_PBCControl.png'))
  PhysicsBasedCameraSensor_1_image : Outport  Tag=outport/plugin/sfun_PBCOutput
  wires:
  Sensor/1 -> PhysicsBasedCameraSensor_1_image/1

== system Test_World_3_cs/PointCloudSensor_1 ==
  Sensor : S-Function  FunctionName=sfun_PCS  Parameters=sensorID, dataWidth, dataHeight, numChannels, dataType, timestep  SFunctionDeploymentMode=off  EnableBusSupport=off  mask(PreScan Source Block: Point Cloud Sensor){sensorID=9052, dataWidth=16, dataHeight=900, numChannels=4, dataType=0, timestep=1/20}
      mask prompts: sensorID "Sensor ID"; dataWidth "Data Width"; dataHeight "Data Height"; numChannels "Channel Count"; dataType "Data Type"; timestep "MATLAB timestep:"
      mask help: The Point Cloud Sensor provides XYZ positions relative to the sensor
      mask Help: eval('openHelp(6400)')
      mask Display: image(imread('PointCloudSensorSL.png'))
  PointCloudSensor_1 : Outport  Tag=outport/PointCloudInport  OutDataTypeStr=single  SampleTime=1/20
  wires:
  Sensor/1 -> PointCloudSensor_1/1
